simulink library "lib_rfsignalgenerator_2020a"  (R2020a)
settings: Solver=VariableStepAuto  StartTime=0.0  StopTime=10.0  RelTol=1e-3
undefined symbols (not defined in the file or in its folder): fs, QAM1024_Sym, QAM512_Sym
libraries: hdlsllib x41, simulink x15, commseqgen3 x10
(part 1 of 2)
settings Model: Creator=lewisdav  LastModifiedBy=bin
settings SFSimCC: CustomCodeUndefinedFunction=UseInterfaceOnly

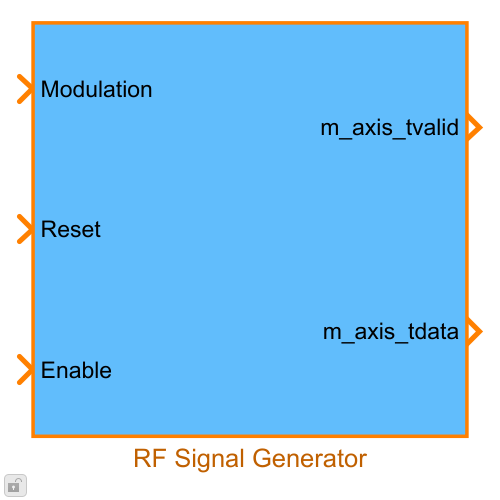
[thumbnail: Simulink's stored preview of the top-level diagram]
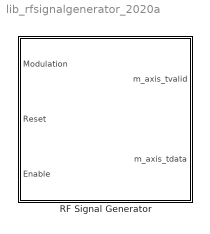
== system lib_rfsignalgenerator_2020a ==
  RF Signal Generator : Subsystem  TreatAsAtomicUnit=on

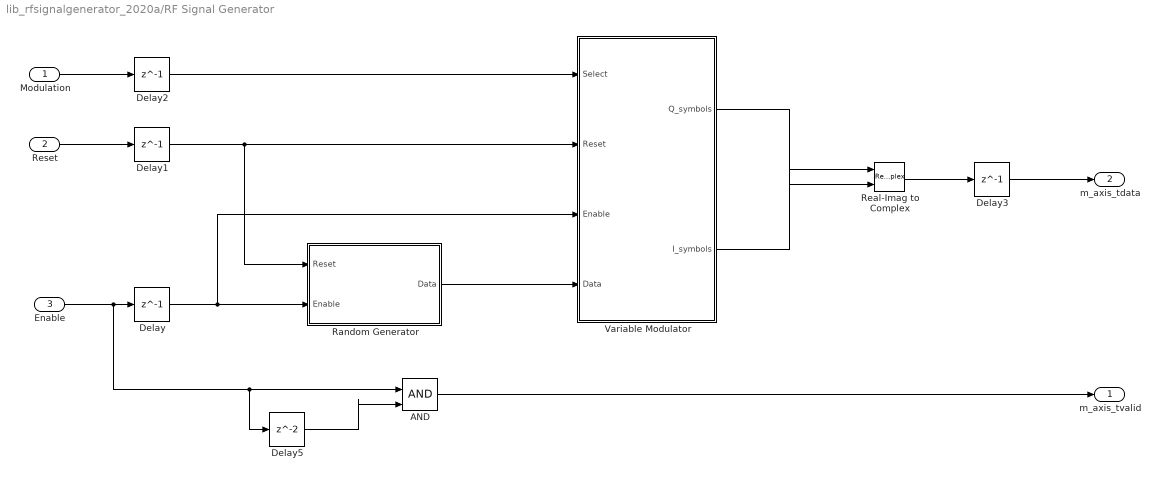
== system lib_rfsignalgenerator_2020a/RF Signal Generator ==
  Modulation : Inport
  Reset : Inport  Port=2
  Enable : Inport  Port=3
  AND : Logic  IconShape=distinctive  AllPortsSameDT=off  OutDataTypeStr=boolean
  Delay{,1..3} (4 alike) : Delay  DelayLength=1
  Delay5 : Delay
  Random Generator : Subsystem
  Real-Imag to Complex : RealImagToComplex
  Variable Modulator : Subsystem
  m_axis_tvalid : Outport  VectorParamsAs1DForOutWhenUnconnected=off
  m_axis_tdata : Outport  Port=2  VectorParamsAs1DForOutWhenUnconnected=off
  wires:
  Delay/1 -> Variable Modulator/3(Enable), Random Generator/2(Enable)
  Random Generator/1(Data) -> Variable Modulator/4(Data)
  Real-Imag to Complex/1 -> Delay3/1
  Modulation/1 -> Delay2/1
  Reset/1 -> Delay1/1
  Enable/1 -> Delay5/1, AND/1, Delay/1
  Delay1/1 -> Variable Modulator/2(Reset), Random Generator/1(Reset)
  Delay2/1 -> Variable Modulator/1(Select)
  Delay3/1 -> m_axis_tdata/1
  AND/1 -> m_axis_tvalid/1
  Variable Modulator/1(Q_symbols) -> Real-Imag to Complex/2
  Variable Modulator/2(I_symbols) -> Real-Imag to Complex/1
  Delay5/1 -> AND/2

== system lib_rfsignalgenerator_2020a/RF Signal Generator/Random Generator ==
  Reset : Inport
  Enable : Inport  Port=2
  Bit Concat1 : hdlsllib/Logic and Bit Operations/Bit Concat  numInputs=10
  Delay : Delay  DelayLength=1  ExternalReset=Level  ShowEnablePort=on  SampleTime=1/fs
      settings: InputPortMap=u0,e6,r5
  Subsystem : Subsystem
  Data : Outport  VectorParamsAs1DForOutWhenUnconnected=off
  wires:
  Enable/1 -> Subsystem/Enable, Delay/2
  Delay/1 -> Data/1
  Bit Concat1/1 -> Delay/1
  Reset/1 -> Delay/3, Subsystem/1(Reset)
  Subsystem/1(LFSR1) -> Bit Concat1/1
  Subsystem/2(LFSR2) -> Bit Concat1/2
  Subsystem/3(LFSR3) -> Bit Concat1/3
  Subsystem/4(LFSR4) -> Bit Concat1/4
  Subsystem/5(LFSR5) -> Bit Concat1/5
  Subsystem/6(LFSR6) -> Bit Concat1/6
  Subsystem/7(LFSR7) -> Bit Concat1/7
  Subsystem/8(LFSR8) -> Bit Concat1/8
  Subsystem/9(LFSR9) -> Bit Concat1/9
  Subsystem/10(LFSR10) -> Bit Concat1/10

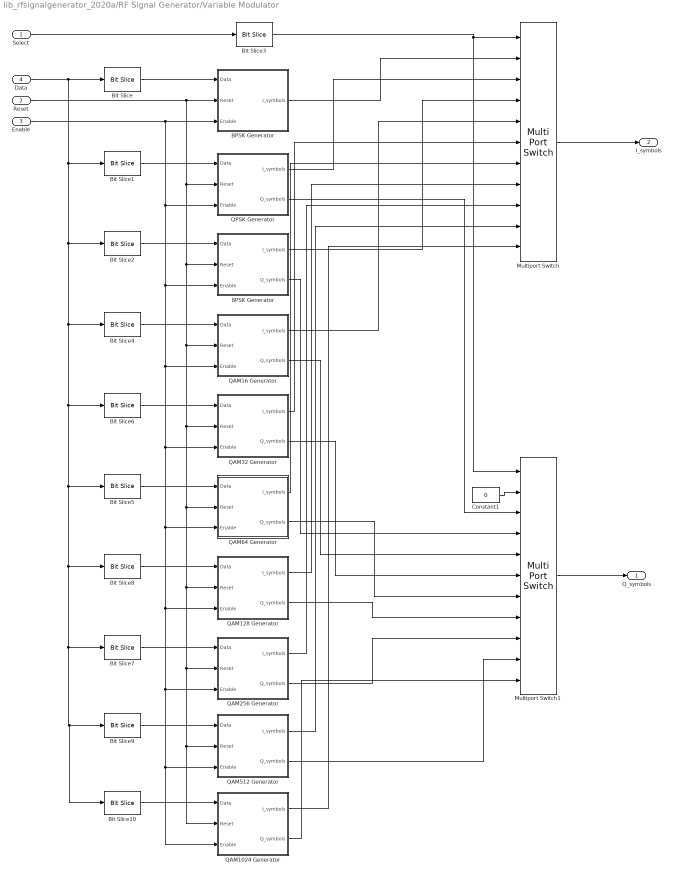
== system lib_rfsignalgenerator_2020a/RF Signal Generator/Variable Modulator ==
  Select : Inport
  Reset : Inport  Port=2
  Enable : Inport  Port=3
  Data : Inport  Port=4
  8PSK Generator : Subsystem
  BPSK Generator : Subsystem
  Bit Slice : hdlsllib/Logic and Bit Operations/Bit Slice  lidx=0  ridx=0
      settings: SourceProductBaseCode=SL
  Bit Slice1 : hdlsllib/Logic and Bit Operations/Bit Slice  lidx=1  ridx=0
      settings: SourceProductBaseCode=SL
  Bit Slice10 : hdlsllib/Logic and Bit Operations/Bit Slice  lidx=9  ridx=0
      settings: SourceProductBaseCode=SL
  Bit Slice2 : hdlsllib/Logic and Bit Operations/Bit Slice  lidx=2  ridx=0
      settings: SourceProductBaseCode=SL
  Bit Slice3 : hdlsllib/Logic and Bit Operations/Bit Slice  lidx=3  ridx=0
      settings: SourceProductBaseCode=SL
  Bit Slice4 : hdlsllib/Logic and Bit Operations/Bit Slice  lidx=3  ridx=0
      settings: SourceProductBaseCode=SL
  Bit Slice5 : hdlsllib/Logic and Bit Operations/Bit Slice  lidx=5  ridx=0
      settings: SourceProductBaseCode=SL
  Bit Slice6 : hdlsllib/Logic and Bit Operations/Bit Slice  lidx=4  ridx=0
      settings: SourceProductBaseCode=SL
  Bit Slice7 : hdlsllib/Logic and Bit Operations/Bit Slice  lidx=7  ridx=0
      settings: SourceProductBaseCode=SL
  Bit Slice8 : hdlsllib/Logic and Bit Operations/Bit Slice  lidx=6  ridx=0
      settings: SourceProductBaseCode=SL
  Bit Slice9 : hdlsllib/Logic and Bit Operations/Bit Slice  lidx=8  ridx=0
      settings: SourceProductBaseCode=SL
  Constant1 : Constant  Value=0  VectorParams1D=off  OutDataTypeStr=fixdt(0,1,0)  SampleTime=1/fs
  Multiport Switch : MultiPortSwitch  DataPortOrder=Zero-based contiguous  Inputs=10  zeroidx=on
  Multiport Switch1 : MultiPortSwitch  DataPortOrder=Zero-based contiguous  Inputs=10  zeroidx=on
  QAM1024 Generator : Subsystem
  QAM128 Generator : Subsystem
  QAM16 Generator : Subsystem
  QAM256 Generator : Subsystem
  QAM32 Generator : Subsystem
  QAM512 Generator : Subsystem
  QAM64 Generator : Subsystem
  QPSK Generator : Subsystem
  Q_symbols : Outport  VectorParamsAs1DForOutWhenUnconnected=off
  I_symbols : Outport  Port=2  VectorParamsAs1DForOutWhenUnconnected=off
  wires:
  QAM512 Generator/2(Q_symbols) -> Multiport Switch1/10
  QAM512 Generator/1(I_symbols) -> Multiport Switch/10
  Bit Slice9/1 -> QAM512 Generator/1(Data)
  Multiport Switch1/1 -> Q_symbols/1
  Multiport Switch/1 -> I_symbols/1
  QAM16 Generator/2(Q_symbols) -> Multiport Switch1/5
  QAM16 Generator/1(I_symbols) -> Multiport Switch/5
  8PSK Generator/2(Q_symbols) -> Multiport Switch1/4
  8PSK Generator/1(I_symbols) -> Multiport Switch/4
  Data/1 -> Bit Slice/1, Bit Slice1/1, Bit Slice2/1, Bit Slice5/1, Bit Slice8/1, Bit Slice7/1, Bit Slice10/1, Bit Slice9/1, Bit Slice6/1, Bit Slice4/1
  QPSK Generator/2(Q_symbols) -> Multiport Switch1/3
  QPSK Generator/1(I_symbols) -> Multiport Switch/3
  Reset/1 -> 8PSK Generator/2(Reset), QAM64 Generator/2(Reset), QAM256 Generator/2(Reset), QAM1024 Generator/2(Reset), QAM512 Generator/2(Reset), QAM128 Generator/2(Reset), QAM32 Generator/2(Reset), QAM16 Generator/2(Reset), QPSK Generator/2(Reset), BPSK Generator/2(Reset)
  Enable/1 -> BPSK Generator/3(Enable), QPSK Generator/3(Enable), 8PSK Generator/3(Enable), QAM64 Generator/3(Enable), QAM256 Generator/3(Enable), QAM1024 Generator/3(Enable), QAM512 Generator/3(Enable), QAM128 Generator/3(Enable), QAM32 Generator/3(Enable), QAM16 Generator/3(Enable)
  BPSK Generator/1(I_symbols) -> Multiport Switch/2
  Bit Slice1/1 -> QPSK Generator/1(Data)
  Select/1 -> Bit Slice3/1
  Bit Slice2/1 -> 8PSK Generator/1(Data)
  Bit Slice/1 -> BPSK Generator/1(Data)
  Constant1/1 -> Multiport Switch1/2
  Bit Slice3/1 -> Multiport Switch/1, Multiport Switch1/1
  Bit Slice4/1 -> QAM16 Generator/1(Data)
  Bit Slice5/1 -> QAM64 Generator/1(Data)
  QAM64 Generator/1(I_symbols) -> Multiport Switch/7
  QAM64 Generator/2(Q_symbols) -> Multiport Switch1/7
  Bit Slice6/1 -> QAM32 Generator/1(Data)
  QAM32 Generator/1(I_symbols) -> Multiport Switch/6
  QAM32 Generator/2(Q_symbols) -> Multiport Switch1/6
  Bit Slice7/1 -> QAM256 Generator/1(Data)
  QAM256 Generator/1(I_symbols) -> Multiport Switch/9
  QAM256 Generator/2(Q_symbols) -> Multiport Switch1/9
  Bit Slice8/1 -> QAM128 Generator/1(Data)
  QAM128 Generator/1(I_symbols) -> Multiport Switch/8
  QAM128 Generator/2(Q_symbols) -> Multiport Switch1/8
  Bit Slice10/1 -> QAM1024 Generator/1(Data)
  QAM1024 Generator/2(Q_symbols) -> Multiport Switch1/11
  QAM1024 Generator/1(I_symbols) -> Multiport Switch/11

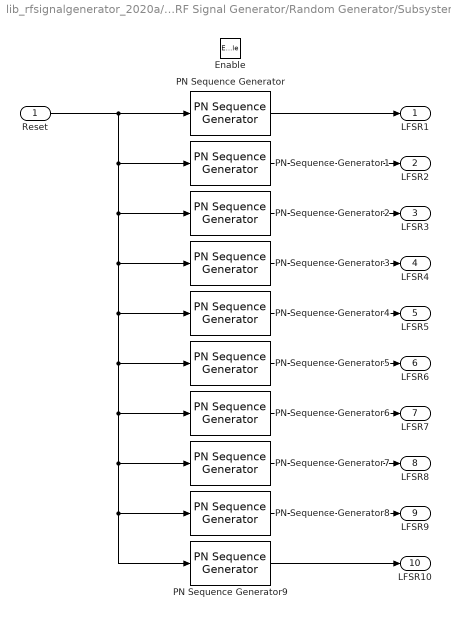
== system lib_rfsignalgenerator_2020a/RF Signal Generator/Random Generator/Subsystem ==
  Reset : Inport
  Enable : EnablePort
  PN Sequence Generator : commseqgen3/PN Sequence Generator  poly='z^13 + z^12 + z^11 + z^8 + 1'  ini_sta=[0 1 1 0 0 0 0 0 0 1 0 0 0]  outBitMaskSource=Dialog parameter  shift=0  outVarSiz=off  maxOutSizeMode=Dialog parameter  maxOutSize=[10 1]  Ts=1/fs  sampPerFrame=1  reset=on  bitPackedOutputs=off  outDataType=boolean  numPackedBits=8  bitPackDataSigned=off  bitPackedOutDType=Smallest integer
  PN Sequence Generator1 : commseqgen3/PN Sequence Generator  poly='z^13 + z^12 + z^11 + z^8 + 1'  ini_sta=[0 0 1 1 0 0 0 0 0 0 0 1 1]  outBitMaskSource=Dialog parameter  shift=0  outVarSiz=off  maxOutSizeMode=Dialog parameter  maxOutSize=[10 1]  Ts=1/fs  sampPerFrame=1  reset=on  bitPackedOutputs=off  outDataType=boolean  numPackedBits=8  bitPackDataSigned=off  bitPackedOutDType=Smallest integer
  PN Sequence Generator2 : commseqgen3/PN Sequence Generator  poly='z^13 + z^12 + z^11 + z^8 + 1'  ini_sta=[1 1 0 1 0 0 0 0 0 1 0 0 1]  outBitMaskSource=Dialog parameter  shift=0  outVarSiz=off  maxOutSizeMode=Dialog parameter  maxOutSize=[10 1]  Ts=1/fs  sampPerFrame=1  reset=on  bitPackedOutputs=off  outDataType=boolean  numPackedBits=8  bitPackDataSigned=off  bitPackedOutDType=Smallest integer
  PN Sequence Generator3 : commseqgen3/PN Sequence Generator  poly='z^13 + z^12 + z^11 + z^8 + 1'  ini_sta=[1 0 1 0 0 0 0 1 0 0 1 1 0]  outBitMaskSource=Dialog parameter  shift=0  outVarSiz=off  maxOutSizeMode=Dialog parameter  maxOutSize=[10 1]  Ts=1/fs  sampPerFrame=1  reset=on  bitPackedOutputs=off  outDataType=boolean  numPackedBits=8  bitPackDataSigned=off  bitPackedOutDType=Smallest integer
  PN Sequence Generator4 : commseqgen3/PN Sequence Generator  poly='z^13 + z^12 + z^11 + z^8 + 1'  ini_sta=[0 0 0 0 1 0 0 0 0 1 1 1 0]  outBitMaskSource=Dialog parameter  shift=0  outVarSiz=off  maxOutSizeMode=Dialog parameter  maxOutSize=[10 1]  Ts=1/fs  sampPerFrame=1  reset=on  bitPackedOutputs=off  outDataType=boolean  numPackedBits=8  bitPackDataSigned=off  bitPackedOutDType=Smallest integer
  PN Sequence Generator5 : commseqgen3/PN Sequence Generator  poly='z^13 + z^12 + z^11 + z^8 + 1'  ini_sta=[1 1 0 0 1 1 0 0 1 0 1 0 0]  outBitMaskSource=Dialog parameter  shift=0  outVarSiz=off  maxOutSizeMode=Dialog parameter  maxOutSize=[10 1]  Ts=1/fs  sampPerFrame=1  reset=on  bitPackedOutputs=off  outDataType=boolean  numPackedBits=8  bitPackDataSigned=off  bitPackedOutDType=Smallest integer
  PN Sequence Generator6 : commseqgen3/PN Sequence Generator  poly='z^13 + z^12 + z^11 + z^8 + 1'  ini_sta=[1 0 0 0 0 1 0 0 0 0 1 1 1]  outBitMaskSource=Dialog parameter  shift=0  outVarSiz=off  maxOutSizeMode=Dialog parameter  maxOutSize=[10 1]  Ts=1/fs  sampPerFrame=1  reset=on  bitPackedOutputs=off  outDataType=boolean  numPackedBits=8  bitPackDataSigned=off  bitPackedOutDType=Smallest integer
  PN Sequence Generator7 : commseqgen3/PN Sequence Generator  poly='z^13 + z^12 + z^11 + z^8 + 1'  ini_sta=[1 0 0 1 1 1 1 1 0 0 0 1 1]  outBitMaskSource=Dialog parameter  shift=0  outVarSiz=off  maxOutSizeMode=Dialog parameter  maxOutSize=[10 1]  Ts=1/fs  sampPerFrame=1  reset=on  bitPackedOutputs=off  outDataType=boolean  numPackedBits=8  bitPackDataSigned=off  bitPackedOutDType=Smallest integer
  PN Sequence Generator8 : commseqgen3/PN Sequence Generator  poly='z^13 + z^12 + z^11 + z^8 + 1'  ini_sta=[1 1 0 1 1 1 1 1 0 0 0 1 1]  outBitMaskSource=Dialog parameter  shift=0  outVarSiz=off  maxOutSizeMode=Dialog parameter  maxOutSize=[10 1]  Ts=1/fs  sampPerFrame=1  reset=on  bitPackedOutputs=off  outDataType=boolean  numPackedBits=8  bitPackDataSigned=off  bitPackedOutDType=Smallest integer
  PN Sequence Generator9 : commseqgen3/PN Sequence Generator  poly='z^13 + z^12 + z^11 + z^8 + 1'  ini_sta=[0 1 0 1 1 0 0 1 0 0 0 1 1]  outBitMaskSource=Dialog parameter  shift=0  outVarSiz=off  maxOutSizeMode=Dialog parameter  maxOutSize=[10 1]  Ts=1/fs  sampPerFrame=1  reset=on  bitPackedOutputs=off  outDataType=boolean  numPackedBits=8  bitPackDataSigned=off  bitPackedOutDType=Smallest integer
  LFSR1 : Outport  InitialOutput=0
  LFSR2 : Outport  Port=2  InitialOutput=0
  LFSR3 : Outport  Port=3  InitialOutput=0
  LFSR4 : Outport  Port=4  InitialOutput=0
  LFSR5 : Outport  Port=5  InitialOutput=0
  LFSR6 : Outport  Port=6  InitialOutput=0
  LFSR7 : Outport  Port=7  InitialOutput=0
  LFSR8 : Outport  Port=8  InitialOutput=0
  LFSR9 : Outport  Port=9  InitialOutput=0
  LFSR10 : Outport  Port=10  InitialOutput=0
  wires:
  PN Sequence Generator8/1 -> LFSR9/1
  PN Sequence Generator/1 -> LFSR1/1
  Reset/1 -> PN Sequence Generator1/1, PN Sequence Generator4/1, PN Sequence Generator5/1, PN Sequence Generator6/1, PN Sequence Generator7/1, PN Sequence Generator9/1, PN Sequence Generator8/1, PN Sequence Generator3/1, PN Sequence Generator2/1, PN Sequence Generator/1
  PN Sequence Generator3/1 -> LFSR4/1
  PN Sequence Generator4/1 -> LFSR5/1
  PN Sequence Generator1/1 -> LFSR2/1
  PN Sequence Generator2/1 -> LFSR3/1
  PN Sequence Generator5/1 -> LFSR6/1
  PN Sequence Generator6/1 -> LFSR7/1
  PN Sequence Generator7/1 -> LFSR8/1
  PN Sequence Generator9/1 -> LFSR10/1

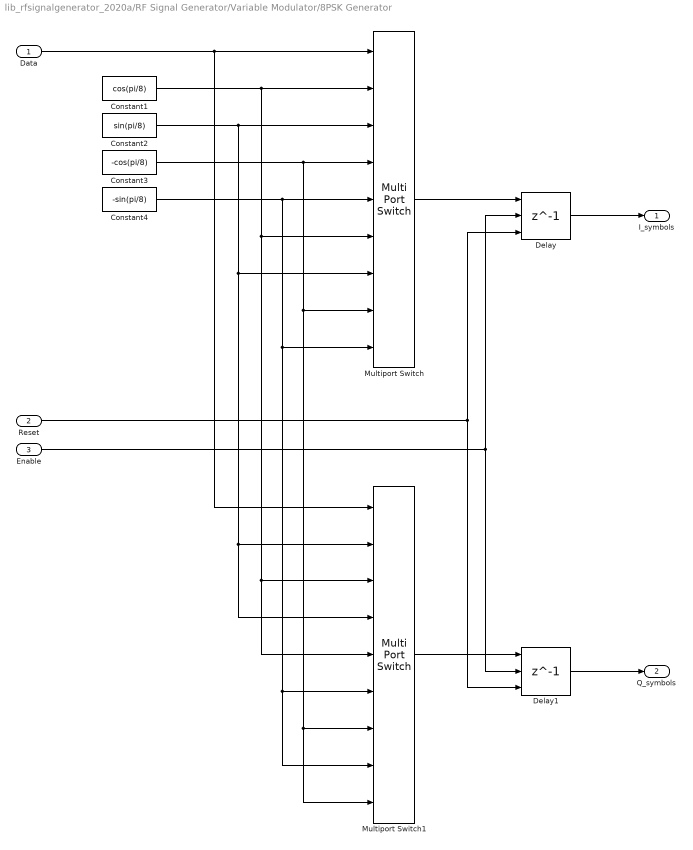
== system lib_rfsignalgenerator_2020a/RF Signal Generator/Variable Modulator/8PSK Generator ==
  Data : Inport
  Reset : Inport  Port=2
  Enable : Inport  Port=3
  Constant1 : Constant  Value=cos(pi/8)  OutDataTypeStr=fixdt(1,16,14)  SampleTime=1/fs
  Constant2 : Constant  Value=sin(pi/8)  VectorParams1D=off  OutDataTypeStr=fixdt(1,16,14)  SampleTime=1/fs
  Constant3 : Constant  Value=-cos(pi/8)  OutDataTypeStr=fixdt(1,16,14)  SampleTime=1/fs
  Constant4 : Constant  Value=-sin(pi/8)  OutDataTypeStr=fixdt(1,16,14)  SampleTime=1/fs
  Delay : Delay  DelayLength=1  ExternalReset=Level  ShowEnablePort=on  SampleTime=1/fs
      settings: InputPortMap=u0,e6,r5
  Delay1 : Delay  DelayLength=1  ExternalReset=Level  ShowEnablePort=on  SampleTime=1/fs
      settings: InputPortMap=u0,e6,r5
  Multiport Switch : MultiPortSwitch  DataPortOrder=Zero-based contiguous  Inputs=8  zeroidx=on
  Multiport Switch1 : MultiPortSwitch  DataPortOrder=Zero-based contiguous  Inputs=8  zeroidx=on
  I_symbols : Outport  VectorParamsAs1DForOutWhenUnconnected=off
  Q_symbols : Outport  Port=2  VectorParamsAs1DForOutWhenUnconnected=off
  wires:
  Delay/1 -> I_symbols/1
  Data/1 -> Multiport Switch/1, Multiport Switch1/1
  Multiport Switch/1 -> Delay/1
  Reset/1 -> Delay/3, Delay1/3
  Enable/1 -> Delay/2, Delay1/2
  Multiport Switch1/1 -> Delay1/1
  Delay1/1 -> Q_symbols/1
  Constant1/1 -> Multiport Switch1/3, Multiport Switch1/5, Multiport Switch/6, Multiport Switch/2
  Constant2/1 -> Multiport Switch1/4, Multiport Switch1/2, Multiport Switch/7, Multiport Switch/3
  Constant3/1 -> Multiport Switch1/7, Multiport Switch1/9, Multiport Switch/8, Multiport Switch/4
  Constant4/1 -> Multiport Switch1/8, Multiport Switch1/6, Multiport Switch/9, Multiport Switch/5

== system lib_rfsignalgenerator_2020a/RF Signal Generator/Variable Modulator/BPSK Generator ==
  Data : Inport
  Reset : Inport  Port=2
  Enable : Inport  Port=3
  Constant2 : Constant  OutDataTypeStr=fixdt(1,16,14)  SampleTime=1/fs
  Constant3 : Constant  Value=-1  OutDataTypeStr=fixdt(1,16,14)  SampleTime=1/fs
  Delay : Delay  DelayLength=1  InitialCondition=0  ExternalReset=Level  ShowEnablePort=on  UseCircularBuffer=on  SampleTime=1/fs
      settings: InputPortMap=u0,e6,r5
  Multiport Switch : MultiPortSwitch  DataPortOrder=Zero-based contiguous  Inputs=2  zeroidx=on
  I_symbols : Outport  VectorParamsAs1DForOutWhenUnconnected=off
  wires:
  Delay/1 -> I_symbols/1
  Enable/1 -> Delay/2
  Reset/1 -> Delay/3
  Multiport Switch/1 -> Delay/1
  Constant3/1 -> Multiport Switch/2
  Constant2/1 -> Multiport Switch/3
  Data/1 -> Multiport Switch/1

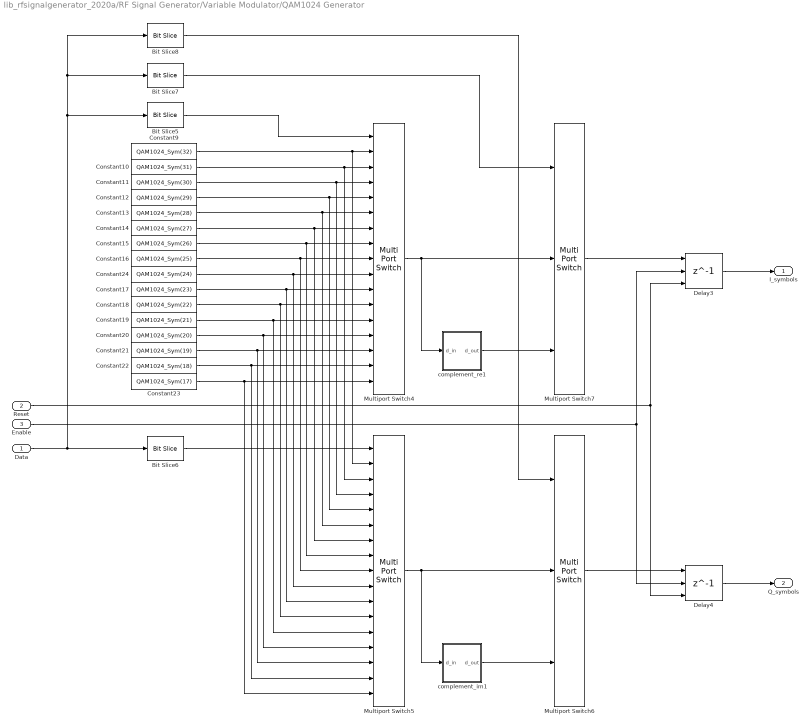
== system lib_rfsignalgenerator_2020a/RF Signal Generator/Variable Modulator/QAM1024 Generator ==
  Data : Inport
  Reset : Inport  Port=2
  Enable : Inport  Port=3
  Bit Slice5 : hdlsllib/Logic and Bit Operations/Bit Slice  lidx=3  ridx=0
      settings: SourceProductBaseCode=SL
  Bit Slice6 : hdlsllib/Logic and Bit Operations/Bit Slice  lidx=7  ridx=4
      settings: SourceProductBaseCode=SL
  Bit Slice7 : hdlsllib/Logic and Bit Operations/Bit Slice  lidx=8  ridx=8
      settings: SourceProductBaseCode=SL
  Bit Slice8 : hdlsllib/Logic and Bit Operations/Bit Slice  lidx=9  ridx=9
      settings: SourceProductBaseCode=SL
  Constant10 : Constant  Value=QAM1024_Sym(31)  OutDataTypeStr=fixdt(1,16,14)  SampleTime=1/fs
  Constant11 : Constant  Value=QAM1024_Sym(30)  OutDataTypeStr=fixdt(1,16,14)  SampleTime=1/fs
  Constant12 : Constant  Value=QAM1024_Sym(29)  OutDataTypeStr=fixdt(1,16,14)  SampleTime=1/fs
  Constant13 : Constant  Value=QAM1024_Sym(28)  OutDataTypeStr=fixdt(1,16,14)  SampleTime=1/fs
  Constant14 : Constant  Value=QAM1024_Sym(27)  OutDataTypeStr=fixdt(1,16,14)  SampleTime=1/fs
  Constant15 : Constant  Value=QAM1024_Sym(26)  OutDataTypeStr=fixdt(1,16,14)  SampleTime=1/fs
  Constant16 : Constant  Value=QAM1024_Sym(25)  OutDataTypeStr=fixdt(1,16,14)  SampleTime=1/fs
  Constant17 : Constant  Value=QAM1024_Sym(23)  OutDataTypeStr=fixdt(1,16,14)  SampleTime=1/fs
  Constant18 : Constant  Value=QAM1024_Sym(22)  OutDataTypeStr=fixdt(1,16,14)  SampleTime=1/fs
  Constant19 : Constant  Value=QAM1024_Sym(21)  OutDataTypeStr=fixdt(1,16,14)  SampleTime=1/fs
  Constant20 : Constant  Value=QAM1024_Sym(20)  OutDataTypeStr=fixdt(1,16,14)  SampleTime=1/fs
  Constant21 : Constant  Value=QAM1024_Sym(19)  OutDataTypeStr=fixdt(1,16,14)  SampleTime=1/fs
  Constant22 : Constant  Value=QAM1024_Sym(18)  OutDataTypeStr=fixdt(1,16,14)  SampleTime=1/fs
  Constant23 : Constant  Value=QAM1024_Sym(17)  OutDataTypeStr=fixdt(1,16,14)  SampleTime=1/fs
  Constant24 : Constant  Value=QAM1024_Sym(24)  OutDataTypeStr=fixdt(1,16,14)  SampleTime=1/fs
  Constant9 : Constant  Value=QAM1024_Sym(32)  OutDataTypeStr=fixdt(1,16,14)  SampleTime=1/fs
  Delay3 : Delay  DelayLength=1  ExternalReset=Level  ShowEnablePort=on  SampleTime=1/fs
      settings: InputPortMap=u0,e6,r5
  Delay4 : Delay  DelayLength=1  ExternalReset=Level  ShowEnablePort=on  SampleTime=1/fs
      settings: InputPortMap=u0,e6,r5
  Multiport Switch4 : MultiPortSwitch  DataPortOrder=Zero-based contiguous  Inputs=16  zeroidx=on
  Multiport Switch5 : MultiPortSwitch  DataPortOrder=Zero-based contiguous  Inputs=16  zeroidx=on
  Multiport Switch6 : MultiPortSwitch  DataPortOrder=Zero-based contiguous  Inputs=2  zeroidx=on
  Multiport Switch7 : MultiPortSwitch  DataPortOrder=Zero-based contiguous  Inputs=2  zeroidx=on
  complement_im1 : Subsystem
  complement_re1 : Subsystem
  I_symbols : Outport  VectorParamsAs1DForOutWhenUnconnected=off
  Q_symbols : Outport  Port=2  VectorParamsAs1DForOutWhenUnconnected=off
  wires:
  Constant9/1 -> Multiport Switch5/2, Multiport Switch4/2
  Constant10/1 -> Multiport Switch5/3, Multiport Switch4/3
  Constant11/1 -> Multiport Switch5/4, Multiport Switch4/4
  Constant13/1 -> Multiport Switch5/6, Multiport Switch4/6
  Constant12/1 -> Multiport Switch5/5, Multiport Switch4/5
  Constant14/1 -> Multiport Switch5/7, Multiport Switch4/7
  Constant15/1 -> Multiport Switch5/8, Multiport Switch4/8
  Constant16/1 -> Multiport Switch5/9, Multiport Switch4/9
  Constant23/1 -> Multiport Switch5/17, Multiport Switch4/17
  Constant22/1 -> Multiport Switch5/16, Multiport Switch4/16
  Constant21/1 -> Multiport Switch5/15, Multiport Switch4/15
  Constant19/1 -> Multiport Switch5/13, Multiport Switch4/13
  Constant18/1 -> Multiport Switch5/12, Multiport Switch4/12
  Constant17/1 -> Multiport Switch5/11, Multiport Switch4/11
  Constant24/1 -> Multiport Switch5/10, Multiport Switch4/10
  Constant20/1 -> Multiport Switch5/14, Multiport Switch4/14
  Multiport Switch5/1 -> Multiport Switch6/2, complement_im1/1(d_in)
  complement_im1/1(d_out) -> Multiport Switch6/3
  Bit Slice7/1 -> Multiport Switch7/1
  Multiport Switch4/1 -> Multiport Switch7/2, complement_re1/1(d_in)
  complement_re1/1(d_out) -> Multiport Switch7/3
  Delay3/1 -> I_symbols/1
  Delay4/1 -> Q_symbols/1
  Reset/1 -> Delay3/3, Delay4/3
  Enable/1 -> Delay3/2, Delay4/2
  Multiport Switch7/1 -> Delay3/1
  Multiport Switch6/1 -> Delay4/1
  Bit Slice5/1 -> Multiport Switch4/1
  Bit Slice6/1 -> Multiport Switch5/1
  Bit Slice8/1 -> Multiport Switch6/1
  Data/1 -> Bit Slice5/1, Bit Slice7/1, Bit Slice8/1, Bit Slice6/1

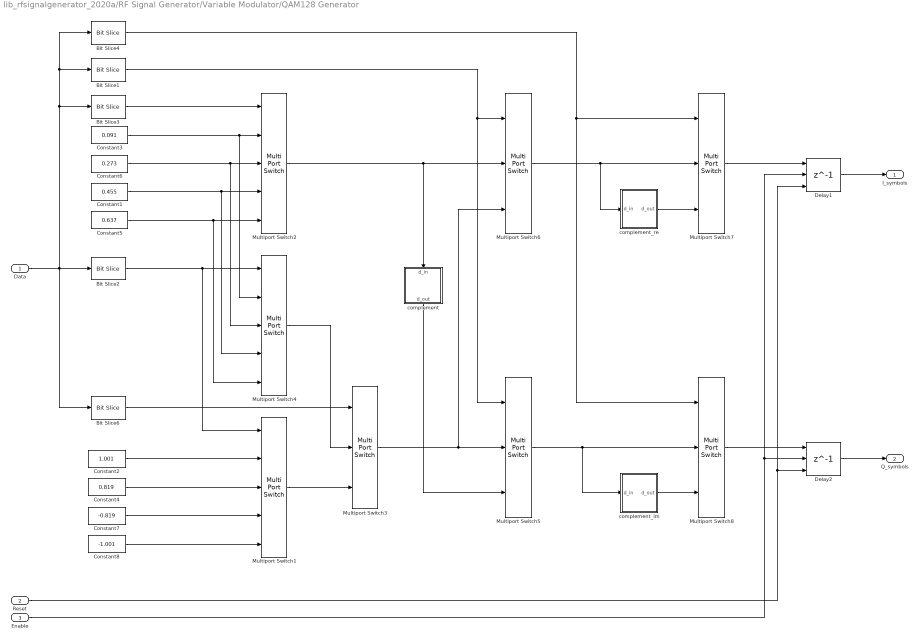
== system lib_rfsignalgenerator_2020a/RF Signal Generator/Variable Modulator/QAM128 Generator ==
  Data : Inport
  Reset : Inport  Port=2
  Enable : Inport  Port=3
  Bit Slice1 : hdlsllib/Logic and Bit Operations/Bit Slice  lidx=5  ridx=5
      settings: SourceProductBaseCode=SL
  Bit Slice2 : hdlsllib/Logic and Bit Operations/Bit Slice  lidx=3  ridx=2
      settings: SourceProductBaseCode=SL
  Bit Slice3 : hdlsllib/Logic and Bit Operations/Bit Slice  lidx=1  ridx=0
      settings: SourceProductBaseCode=SL
  Bit Slice4 : hdlsllib/Logic and Bit Operations/Bit Slice  lidx=6  ridx=6
      settings: SourceProductBaseCode=SL
  Bit Slice6 : hdlsllib/Logic and Bit Operations/Bit Slice  lidx=4  ridx=4
      settings: SourceProductBaseCode=SL
  Constant1 : Constant  Value=0.455  OutDataTypeStr=fixdt(1,16,14)  SampleTime=1/fs
  Constant2 : Constant  Value=1.001  OutDataTypeStr=fixdt(1,16,14)  SampleTime=1/fs
  Constant3 : Constant  Value=0.091  OutDataTypeStr=fixdt(1,16,14)  SampleTime=1/fs
  Constant4 : Constant  Value=0.819  OutDataTypeStr=fixdt(1,16,14)  SampleTime=1/fs
  Constant5 : Constant  Value=0.637  OutDataTypeStr=fixdt(1,16,14)  SampleTime=1/fs
  Constant6 : Constant  Value=0.273  OutDataTypeStr=fixdt(1,16,14)  SampleTime=1/fs
  Constant7 : Constant  Value=-0.819  OutDataTypeStr=fixdt(1,16,14)  SampleTime=1/fs
  Constant8 : Constant  Value=-1.001  OutDataTypeStr=fixdt(1,16,14)  SampleTime=1/fs
  Delay1 : Delay  DelayLength=1  ExternalReset=Level  ShowEnablePort=on  SampleTime=1/fs
      settings: InputPortMap=u0,e6,r5
  Delay2 : Delay  DelayLength=1  ExternalReset=Level  ShowEnablePort=on  SampleTime=1/fs
      settings: InputPortMap=u0,e6,r5
  Multiport Switch1 : MultiPortSwitch  DataPortOrder=Zero-based contiguous  Inputs=4  zeroidx=on
  Multiport Switch2 : MultiPortSwitch  DataPortOrder=Zero-based contiguous  Inputs=4  zeroidx=on
  Multiport Switch{3,5..8} (5 alike) : MultiPortSwitch  DataPortOrder=Zero-based contiguous  Inputs=2  zeroidx=on
  Multiport Switch4 : MultiPortSwitch  DataPortOrder=Zero-based contiguous  Inputs=4  zeroidx=on
  complement : Subsystem
  complement_im : Subsystem
  complement_re : Subsystem
  I_symbols : Outport  VectorParamsAs1DForOutWhenUnconnected=off
  Q_symbols : Outport  Port=2  VectorParamsAs1DForOutWhenUnconnected=off
  wires:
  Multiport Switch2/1 -> complement/1(d_in), Multiport Switch6/2
  complement/1(d_out) -> Multiport Switch5/3
  Multiport Switch3/1 -> Multiport Switch5/2, Multiport Switch6/3
  complement_re/1(d_out) -> Multiport Switch7/3
  complement_im/1(d_out) -> Multiport Switch8/3
  Bit Slice4/1 -> Multiport Switch7/1, Multiport Switch8/1
  Bit Slice1/1 -> Multiport Switch6/1, Multiport Switch5/1
  Multiport Switch8/1 -> Delay2/1
  Multiport Switch7/1 -> Delay1/1
  Multiport Switch5/1 -> complement_im/1(d_in), Multiport Switch8/2
  Multiport Switch6/1 -> complement_re/1(d_in), Multiport Switch7/2
  Bit Slice6/1 -> Multiport Switch3/1
  Multiport Switch1/1 -> Multiport Switch3/3
  Constant8/1 -> Multiport Switch1/5
  Constant7/1 -> Multiport Switch1/4
  Constant5/1 -> Multiport Switch2/5, Multiport Switch4/5
  Constant1/1 -> Multiport Switch2/4, Multiport Switch4/4
  Multiport Switch4/1 -> Multiport Switch3/2
  Data/1 -> Bit Slice3/1, Bit Slice1/1, Bit Slice4/1, Bit Slice6/1, Bit Slice2/1
  Enable/1 -> Delay1/2, Delay2/2
  Reset/1 -> Delay1/3, Delay2/3
  Constant2/1 -> Multiport Switch1/2
  Constant4/1 -> Multiport Switch1/3
  Delay2/1 -> Q_symbols/1
  Delay1/1 -> I_symbols/1
  Constant3/1 -> Multiport Switch2/2, Multiport Switch4/2
  Constant6/1 -> Multiport Switch2/3, Multiport Switch4/3
  Bit Slice3/1 -> Multiport Switch2/1
  Bit Slice2/1 -> Multiport Switch4/1, Multiport Switch1/1

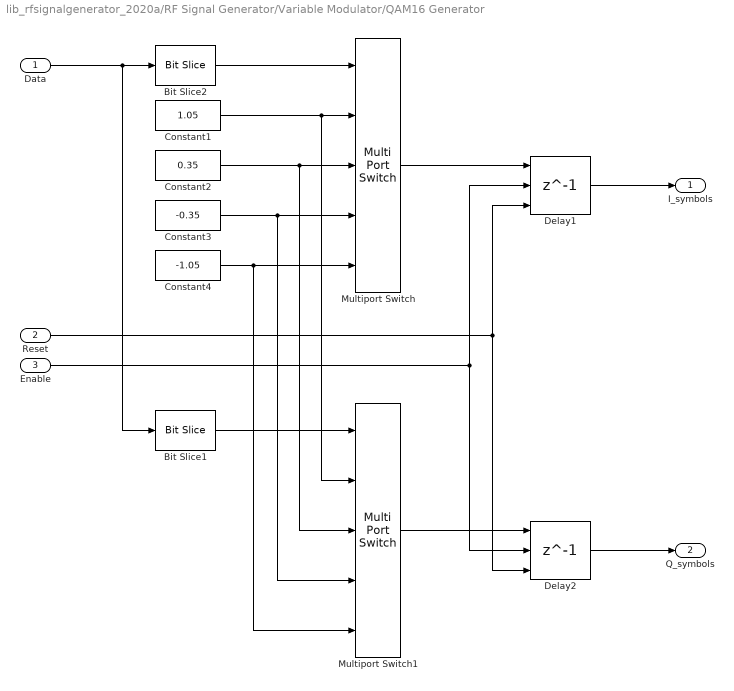
== system lib_rfsignalgenerator_2020a/RF Signal Generator/Variable Modulator/QAM16 Generator ==
  Data : Inport
  Reset : Inport  Port=2
  Enable : Inport  Port=3
  Bit Slice1 : hdlsllib/Logic and Bit Operations/Bit Slice  lidx=3  ridx=2
      settings: SourceProductBaseCode=SL
  Bit Slice2 : hdlsllib/Logic and Bit Operations/Bit Slice  lidx=1  ridx=0
      settings: SourceProductBaseCode=SL
  Constant1 : Constant  Value=1.05  OutDataTypeStr=fixdt(1,16,14)  SampleTime=1/fs
  Constant2 : Constant  Value=0.35  OutDataTypeStr=fixdt(1,16,14)  SampleTime=1/fs
  Constant3 : Constant  Value=-0.35  OutDataTypeStr=fixdt(1,16,14)  SampleTime=1/fs
  Constant4 : Constant  Value=-1.05  OutDataTypeStr=fixdt(1,16,14)  SampleTime=1/fs
  Delay1 : Delay  DelayLength=1  ExternalReset=Level  ShowEnablePort=on  SampleTime=1/fs
      settings: InputPortMap=u0,e6,r5
  Delay2 : Delay  DelayLength=1  ExternalReset=Level  ShowEnablePort=on  SampleTime=1/fs
      settings: InputPortMap=u0,e6,r5
  Multiport Switch : MultiPortSwitch  DataPortOrder=Zero-based contiguous  Inputs=4  zeroidx=on
  Multiport Switch1 : MultiPortSwitch  DataPortOrder=Zero-based contiguous  Inputs=4  zeroidx=on
  I_symbols : Outport  VectorParamsAs1DForOutWhenUnconnected=off
  Q_symbols : Outport  Port=2  VectorParamsAs1DForOutWhenUnconnected=off
  wires:
  Data/1 -> Bit Slice2/1, Bit Slice1/1
  Bit Slice2/1 -> Multiport Switch/1
  Multiport Switch/1 -> Delay1/1
  Delay1/1 -> I_symbols/1
  Multiport Switch1/1 -> Delay2/1
  Delay2/1 -> Q_symbols/1
  Reset/1 -> Delay1/3, Delay2/3
  Enable/1 -> Delay1/2, Delay2/2
  Bit Slice1/1 -> Multiport Switch1/1
  Constant1/1 -> Multiport Switch/2, Multiport Switch1/2
  Constant2/1 -> Multiport Switch/3, Multiport Switch1/3
  Constant3/1 -> Multiport Switch/4, Multiport Switch1/4
  Constant4/1 -> Multiport Switch/5, Multiport Switch1/5

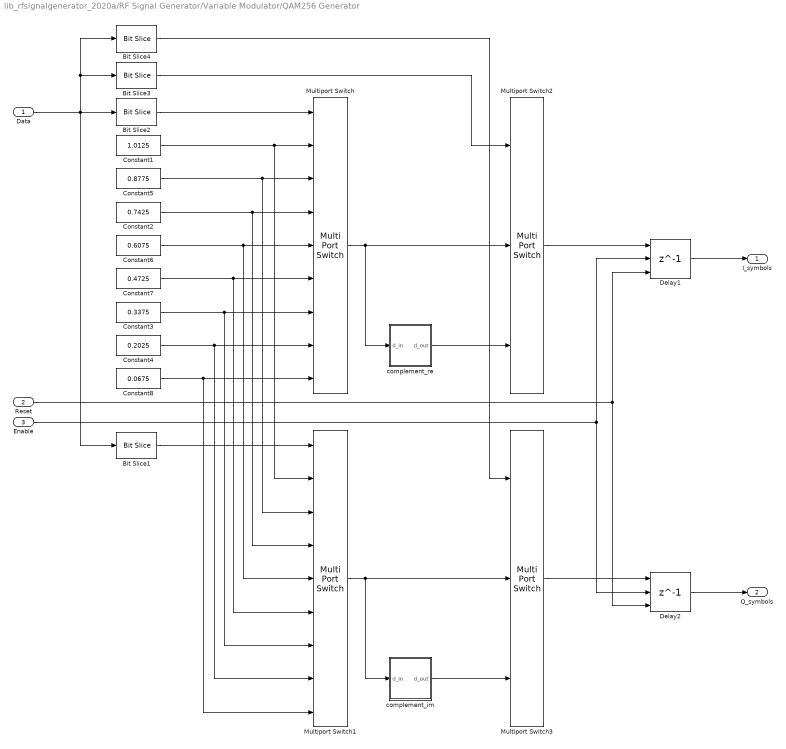
== system lib_rfsignalgenerator_2020a/RF Signal Generator/Variable Modulator/QAM256 Generator ==
  Data : Inport
  Reset : Inport  Port=2
  Enable : Inport  Port=3
  Bit Slice1 : hdlsllib/Logic and Bit Operations/Bit Slice  lidx=5  ridx=3
      settings: SourceProductBaseCode=SL
  Bit Slice2 : hdlsllib/Logic and Bit Operations/Bit Slice  lidx=2  ridx=0
      settings: SourceProductBaseCode=SL
  Bit Slice3 : hdlsllib/Logic and Bit Operations/Bit Slice  lidx=6  ridx=6
      settings: SourceProductBaseCode=SL
  Bit Slice4 : hdlsllib/Logic and Bit Operations/Bit Slice  lidx=7  ridx=7
      settings: SourceProductBaseCode=SL
  Constant1 : Constant  Value=1.0125  OutDataTypeStr=fixdt(1,16,14)  SampleTime=1/fs
  Constant2 : Constant  Value=0.7425  OutDataTypeStr=fixdt(1,16,14)  SampleTime=1/fs
  Constant3 : Constant  Value=0.3375  OutDataTypeStr=fixdt(1,16,14)  SampleTime=1/fs
  Constant4 : Constant  Value=0.2025  OutDataTypeStr=fixdt(1,16,14)  SampleTime=1/fs
  Constant5 : Constant  Value=0.8775  OutDataTypeStr=fixdt(1,16,14)  SampleTime=1/fs
  Constant6 : Constant  Value=0.6075  OutDataTypeStr=fixdt(1,16,14)  SampleTime=1/fs
  Constant7 : Constant  Value=0.4725  OutDataTypeStr=fixdt(1,16,14)  SampleTime=1/fs
  Constant8 : Constant  Value=0.0675  OutDataTypeStr=fixdt(1,16,14)  SampleTime=1/fs
  Delay1 : Delay  DelayLength=1  ExternalReset=Level  ShowEnablePort=on  SampleTime=1/fs
      settings: InputPortMap=u0,e6,r5
  Delay2 : Delay  DelayLength=1  ExternalReset=Level  ShowEnablePort=on  SampleTime=1/fs
      settings: InputPortMap=u0,e6,r5
  Multiport Switch : MultiPortSwitch  DataPortOrder=Zero-based contiguous  Inputs=8  zeroidx=on
  Multiport Switch1 : MultiPortSwitch  DataPortOrder=Zero-based contiguous  Inputs=8  zeroidx=on
  Multiport Switch2 : MultiPortSwitch  DataPortOrder=Zero-based contiguous  Inputs=2  zeroidx=on
  Multiport Switch3 : MultiPortSwitch  DataPortOrder=Zero-based contiguous  Inputs=2  zeroidx=on
  complement_im : Subsystem
  complement_re : Subsystem
  I_symbols : Outport  VectorParamsAs1DForOutWhenUnconnected=off
  Q_symbols : Outport  Port=2  VectorParamsAs1DForOutWhenUnconnected=off
  wires:
  Bit Slice1/1 -> Multiport Switch1/1
  Constant4/1 -> Multiport Switch/8, Multiport Switch1/8
  Constant7/1 -> Multiport Switch/6, Multiport Switch1/6
  Constant6/1 -> Multiport Switch/5, Multiport Switch1/5
  Constant5/1 -> Multiport Switch/3, Multiport Switch1/3
  Constant8/1 -> Multiport Switch/9, Multiport Switch1/9
  Constant3/1 -> Multiport Switch/7, Multiport Switch1/7
  Constant2/1 -> Multiport Switch/4, Multiport Switch1/4
  Data/1 -> Bit Slice2/1, Bit Slice1/1, Bit Slice4/1, Bit Slice3/1
  Bit Slice2/1 -> Multiport Switch/1
  Delay1/1 -> I_symbols/1
  Delay2/1 -> Q_symbols/1
  Reset/1 -> Delay1/3, Delay2/3
  Enable/1 -> Delay2/2, Delay1/2
  Constant1/1 -> Multiport Switch/2, Multiport Switch1/2
  Bit Slice3/1 -> Multiport Switch2/1
  Multiport Switch2/1 -> Delay1/1
  Multiport Switch3/1 -> Delay2/1
  Multiport Switch/1 -> Multiport Switch2/2, complement_re/1(d_in)
  Multiport Switch1/1 -> Multiport Switch3/2, complement_im/1(d_in)
  Bit Slice4/1 -> Multiport Switch3/1
  complement_im/1(d_out) -> Multiport Switch3/3
  complement_re/1(d_out) -> Multiport Switch2/3

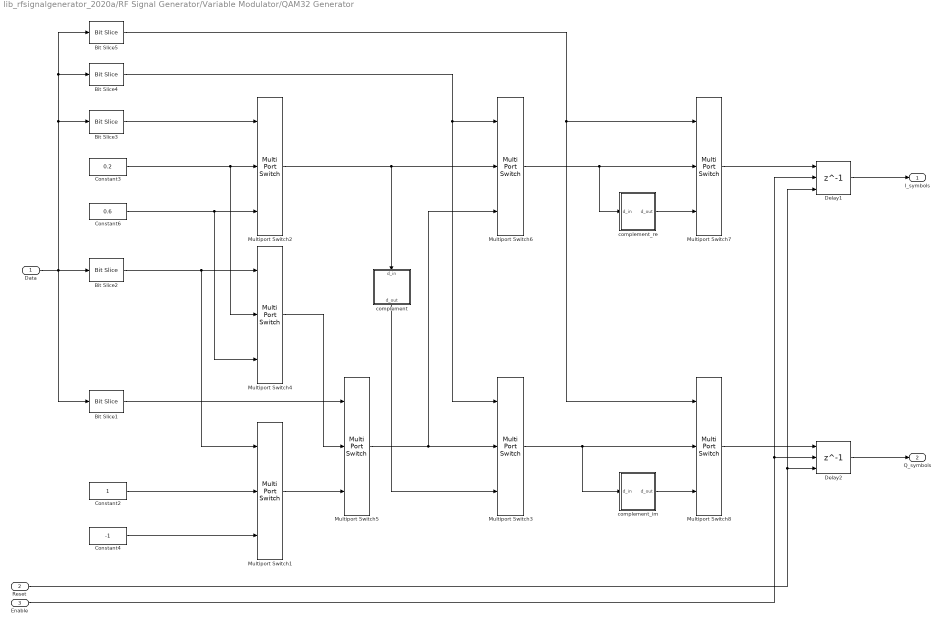
== system lib_rfsignalgenerator_2020a/RF Signal Generator/Variable Modulator/QAM32 Generator ==
  Data : Inport
  Reset : Inport  Port=2
  Enable : Inport  Port=3
  Bit Slice1 : hdlsllib/Logic and Bit Operations/Bit Slice  lidx=2  ridx=2
      settings: SourceProductBaseCode=SL
  Bit Slice2 : hdlsllib/Logic and Bit Operations/Bit Slice  lidx=1  ridx=1
      settings: SourceProductBaseCode=SL
  Bit Slice3 : hdlsllib/Logic and Bit Operations/Bit Slice  lidx=0  ridx=0
      settings: SourceProductBaseCode=SL
  Bit Slice4 : hdlsllib/Logic and Bit Operations/Bit Slice  lidx=3  ridx=3
      settings: SourceProductBaseCode=SL
  Bit Slice5 : hdlsllib/Logic and Bit Operations/Bit Slice  lidx=4  ridx=4
      settings: SourceProductBaseCode=SL
  Constant2 : Constant  OutDataTypeStr=fixdt(1,16,14)  SampleTime=1/fs
  Constant3 : Constant  Value=0.2  OutDataTypeStr=fixdt(1,16,14)  SampleTime=1/fs
  Constant4 : Constant  Value=-1  OutDataTypeStr=fixdt(1,16,14)  SampleTime=1/fs
  Constant6 : Constant  Value=0.6  OutDataTypeStr=fixdt(1,16,14)  SampleTime=1/fs
  Delay1 : Delay  DelayLength=1  ExternalReset=Level  ShowEnablePort=on  SampleTime=1/fs
      settings: InputPortMap=u0,e6,r5
  Delay2 : Delay  DelayLength=1  ExternalReset=Level  ShowEnablePort=on  SampleTime=1/fs
      settings: InputPortMap=u0,e6,r5
  Multiport Switch{1..8} (8 alike) : MultiPortSwitch  DataPortOrder=Zero-based contiguous  Inputs=2  zeroidx=on
  complement : Subsystem
  complement_im : Subsystem
  complement_re : Subsystem
  I_symbols : Outport  VectorParamsAs1DForOutWhenUnconnected=off
  Q_symbols : Outport  Port=2  VectorParamsAs1DForOutWhenUnconnected=off
  wires:
  Data/1 -> Bit Slice5/1, Bit Slice4/1, Bit Slice3/1, Bit Slice1/1, Bit Slice2/1
  Enable/1 -> Delay1/2, Delay2/2
  Reset/1 -> Delay1/3, Delay2/3
  Constant2/1 -> Multiport Switch1/2
  Constant4/1 -> Multiport Switch1/3
  Delay2/1 -> Q_symbols/1
  Delay1/1 -> I_symbols/1
  Constant3/1 -> Multiport Switch4/2, Multiport Switch2/2
  Constant6/1 -> Multiport Switch4/3, Multiport Switch2/3
  Bit Slice3/1 -> Multiport Switch2/1
  Bit Slice2/1 -> Multiport Switch1/1, Multiport Switch4/1
  Multiport Switch4/1 -> Multiport Switch5/2
  Multiport Switch1/1 -> Multiport Switch5/3
  Bit Slice4/1 -> Multiport Switch6/1, Multiport Switch3/1
  Multiport Switch5/1 -> Multiport Switch6/3, Multiport Switch3/2
  Bit Slice5/1 -> Multiport Switch8/1, Multiport Switch7/1
  Multiport Switch6/1 -> Multiport Switch7/2, complement_re/1(d_in)
  Multiport Switch3/1 -> Multiport Switch8/2, complement_im/1(d_in)
  complement/1(d_out) -> Multiport Switch3/3
  complement_re/1(d_out) -> Multiport Switch7/3
  complement_im/1(d_out) -> Multiport Switch8/3
  Multiport Switch2/1 -> Multiport Switch6/2, complement/1(d_in)
  Bit Slice1/1 -> Multiport Switch5/1
  Multiport Switch7/1 -> Delay1/1
  Multiport Switch8/1 -> Delay2/1

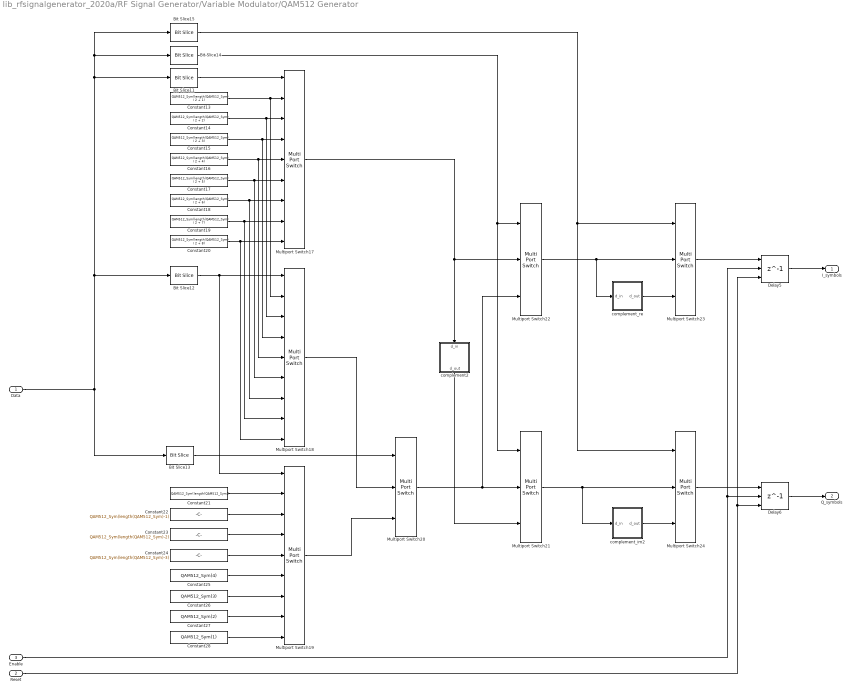
== system lib_rfsignalgenerator_2020a/RF Signal Generator/Variable Modulator/QAM512 Generator ==
  Data : Inport
  Reset : Inport  Port=2
  Enable : Inport  Port=3
  Bit Slice11 : hdlsllib/Logic and Bit Operations/Bit Slice  lidx=2  ridx=0
      settings: SourceProductBaseCode=SL
  Bit Slice12 : hdlsllib/Logic and Bit Operations/Bit Slice  lidx=5  ridx=3
      settings: SourceProductBaseCode=SL
  Bit Slice13 : hdlsllib/Logic and Bit Operations/Bit Slice  lidx=6  ridx=6
      settings: SourceProductBaseCode=SL
  Bit Slice14 : hdlsllib/Logic and Bit Operations/Bit Slice  lidx=7  ridx=7
      settings: SourceProductBaseCode=SL
  Bit Slice15 : hdlsllib/Logic and Bit Operations/Bit Slice  lidx=8  ridx=8
      settings: SourceProductBaseCode=SL
  Constant13 : Constant  Value=QAM512_Sym(length(QAM512_Sym) / 2 + 1)  OutDataTypeStr=fixdt(1,16,14)  SampleTime=1/fs
  Constant14 : Constant  Value=QAM512_Sym(length(QAM512_Sym) / 2 + 2)  OutDataTypeStr=fixdt(1,16,14)  SampleTime=1/fs
  Constant15 : Constant  Value=QAM512_Sym(length(QAM512_Sym) / 2 + 3)  OutDataTypeStr=fixdt(1,16,14)  SampleTime=1/fs
  Constant16 : Constant  Value=QAM512_Sym(length(QAM512_Sym) / 2 + 4)  OutDataTypeStr=fixdt(1,16,14)  SampleTime=1/fs
  Constant17 : Constant  Value=QAM512_Sym(length(QAM512_Sym) / 2 + 5)  OutDataTypeStr=fixdt(1,16,14)  SampleTime=1/fs
  Constant18 : Constant  Value=QAM512_Sym(length(QAM512_Sym) / 2 + 6)  OutDataTypeStr=fixdt(1,16,14)  SampleTime=1/fs
  Constant19 : Constant  Value=QAM512_Sym(length(QAM512_Sym) / 2 + 7)  OutDataTypeStr=fixdt(1,16,14)  SampleTime=1/fs
  Constant20 : Constant  Value=QAM512_Sym(length(QAM512_Sym) / 2 + 8)  OutDataTypeStr=fixdt(1,16,14)  SampleTime=1/fs
  Constant21 : Constant  Value=QAM512_Sym(length(QAM512_Sym))  OutDataTypeStr=fixdt(1,16,14)  SampleTime=1/fs
  Constant22 : Constant  Value=QAM512_Sym(length(QAM512_Sym)-1)  OutDataTypeStr=fixdt(1,16,14)  SampleTime=1/fs
  Constant23 : Constant  Value=QAM512_Sym(length(QAM512_Sym)-2)  OutDataTypeStr=fixdt(1,16,14)  SampleTime=1/fs
  Constant24 : Constant  Value=QAM512_Sym(length(QAM512_Sym)-3)  OutDataTypeStr=fixdt(1,16,14)  SampleTime=1/fs
  Constant25 : Constant  Value=QAM512_Sym(4)  OutDataTypeStr=fixdt(1,16,14)  SampleTime=1/fs
  Constant26 : Constant  Value=QAM512_Sym(3)  OutDataTypeStr=fixdt(1,16,14)  SampleTime=1/fs
  Constant27 : Constant  Value=QAM512_Sym(2)  OutDataTypeStr=fixdt(1,16,14)  SampleTime=1/fs
  Constant28 : Constant  Value=QAM512_Sym(1)  OutDataTypeStr=fixdt(1,16,14)  SampleTime=1/fs
  Delay5 : Delay  DelayLength=1  ExternalReset=Level  ShowEnablePort=on  SampleTime=1/fs
      settings: InputPortMap=u0,e6,r5
  Delay6 : Delay  DelayLength=1  ExternalReset=Level  ShowEnablePort=on  SampleTime=1/fs
      settings: InputPortMap=u0,e6,r5
  Multiport Switch17 : MultiPortSwitch  DataPortOrder=Zero-based contiguous  Inputs=8  zeroidx=on
  Multiport Switch18 : MultiPortSwitch  DataPortOrder=Zero-based contiguous  Inputs=8  zeroidx=on
  Multiport Switch19 : MultiPortSwitch  DataPortOrder=Zero-based contiguous  Inputs=8  zeroidx=on
  Multiport Switch{20..24} (5 alike) : MultiPortSwitch  DataPortOrder=Zero-based contiguous  Inputs=2  zeroidx=on
  complement2 : Subsystem
  complement_im2 : Subsystem
  complement_re : Subsystem
  I_symbols : Outport  VectorParamsAs1DForOutWhenUnconnected=off
  Q_symbols : Outport  Port=2  VectorParamsAs1DForOutWhenUnconnected=off
  wires:
  Constant13/1 -> Multiport Switch18/2, Multiport Switch17/2
  Constant14/1 -> Multiport Switch18/3, Multiport Switch17/3
  Constant15/1 -> Multiport Switch18/4, Multiport Switch17/4
  Constant16/1 -> Multiport Switch18/5, Multiport Switch17/5
  Constant17/1 -> Multiport Switch18/6, Multiport Switch17/6
  Constant18/1 -> Multiport Switch18/7, Multiport Switch17/7
  Constant19/1 -> Multiport Switch18/8, Multiport Switch17/8
  Constant20/1 -> Multiport Switch18/9, Multiport Switch17/9
  Bit Slice11/1 -> Multiport Switch17/1
  Bit Slice12/1 -> Multiport Switch19/1, Multiport Switch18/1
  Constant21/1 -> Multiport Switch19/2
  Constant22/1 -> Multiport Switch19/3
  Constant23/1 -> Multiport Switch19/4
  Constant24/1 -> Multiport Switch19/5
  Constant25/1 -> Multiport Switch19/6
  Constant26/1 -> Multiport Switch19/7
  Constant28/1 -> Multiport Switch19/9
  Constant27/1 -> Multiport Switch19/8
  Multiport Switch18/1 -> Multiport Switch20/2
  Multiport Switch19/1 -> Multiport Switch20/3
  Bit Slice13/1 -> Multiport Switch20/1
  Delay5/1 -> I_symbols/1
  Delay6/1 -> Q_symbols/1
  Reset/1 -> Delay6/3, Delay5/3
  Enable/1 -> Delay6/2, Delay5/2
  Multiport Switch22/1 -> complement_re/1(d_in), Multiport Switch23/2
  Multiport Switch21/1 -> Multiport Switch24/2, complement_im2/1(d_in)
  Multiport Switch23/1 -> Delay5/1
  Multiport Switch24/1 -> Delay6/1
  Bit Slice14/1 -> Multiport Switch21/1, Multiport Switch22/1
  Bit Slice15/1 -> Multiport Switch24/1, Multiport Switch23/1
  complement_im2/1(d_out) -> Multiport Switch24/3
  complement_re/1(d_out) -> Multiport Switch23/3
  Multiport Switch20/1 -> Multiport Switch22/3, Multiport Switch21/2
  complement2/1(d_out) -> Multiport Switch21/3
  Multiport Switch17/1 -> Multiport Switch22/2, complement2/1(d_in)
  Data/1 -> Bit Slice13/1, Bit Slice12/1, Bit Slice11/1, Bit Slice14/1, Bit Slice15/1

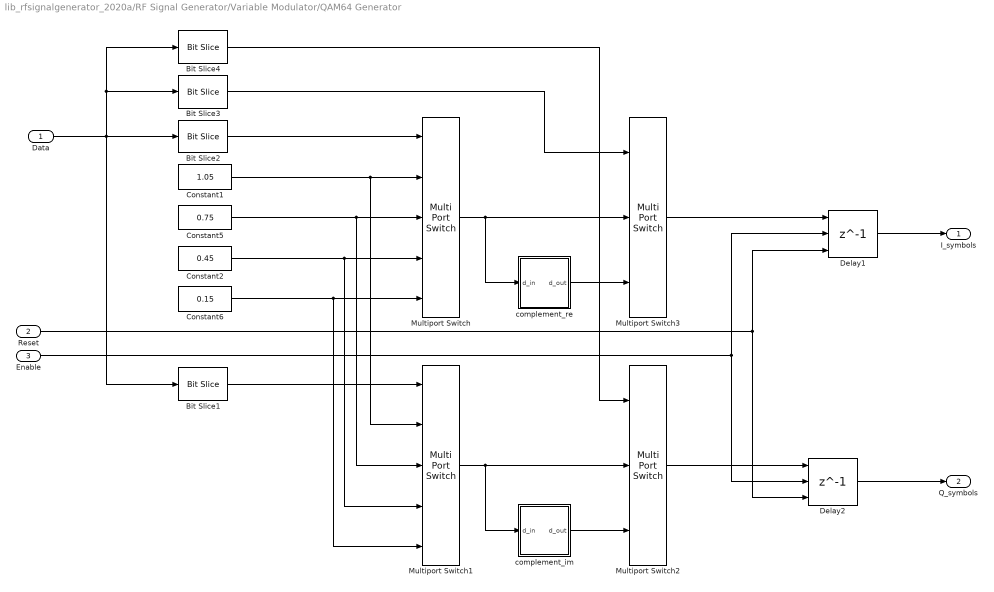
== system lib_rfsignalgenerator_2020a/RF Signal Generator/Variable Modulator/QAM64 Generator ==
  Data : Inport
  Reset : Inport  Port=2
  Enable : Inport  Port=3
  Bit Slice1 : hdlsllib/Logic and Bit Operations/Bit Slice  lidx=3  ridx=2
      settings: SourceProductBaseCode=SL
  Bit Slice2 : hdlsllib/Logic and Bit Operations/Bit Slice  lidx=1  ridx=0
      settings: SourceProductBaseCode=SL
  Bit Slice3 : hdlsllib/Logic and Bit Operations/Bit Slice  lidx=4  ridx=4
      settings: SourceProductBaseCode=SL
  Bit Slice4 : hdlsllib/Logic and Bit Operations/Bit Slice  lidx=5  ridx=5
      settings: SourceProductBaseCode=SL
  Constant1 : Constant  Value=1.05  OutDataTypeStr=fixdt(1,16,14)  SampleTime=1/fs
  Constant2 : Constant  Value=0.45  OutDataTypeStr=fixdt(1,16,14)  SampleTime=1/fs
  Constant5 : Constant  Value=0.75  OutDataTypeStr=fixdt(1,16,14)  SampleTime=1/fs
  Constant6 : Constant  Value=0.15  OutDataTypeStr=fixdt(1,16,14)  SampleTime=1/fs
  Delay1 : Delay  DelayLength=1  ExternalReset=Level  ShowEnablePort=on  SampleTime=1/fs
      settings: InputPortMap=u0,e6,r5
  Delay2 : Delay  DelayLength=1  ExternalReset=Level  ShowEnablePort=on  SampleTime=1/fs
      settings: InputPortMap=u0,e6,r5
  Multiport Switch : MultiPortSwitch  DataPortOrder=Zero-based contiguous  Inputs=4  zeroidx=on
  Multiport Switch1 : MultiPortSwitch  DataPortOrder=Zero-based contiguous  Inputs=4  zeroidx=on
  Multiport Switch2 : MultiPortSwitch  DataPortOrder=Zero-based contiguous  Inputs=2  zeroidx=on
  Multiport Switch3 : MultiPortSwitch  DataPortOrder=Zero-based contiguous  Inputs=2  zeroidx=on
  complement_im : Subsystem
  complement_re : Subsystem
  I_symbols : Outport  VectorParamsAs1DForOutWhenUnconnected=off
  Q_symbols : Outport  Port=2  VectorParamsAs1DForOutWhenUnconnected=off
  wires:
  Constant1/1 -> Multiport Switch1/2, Multiport Switch/2
  Enable/1 -> Delay1/2, Delay2/2
  Reset/1 -> Delay2/3, Delay1/3
  Delay2/1 -> Q_symbols/1
  Delay1/1 -> I_symbols/1
  Bit Slice2/1 -> Multiport Switch/1
  Data/1 -> Bit Slice1/1, Bit Slice4/1, Bit Slice3/1, Bit Slice2/1
  Constant2/1 -> Multiport Switch1/4, Multiport Switch/4
  Constant5/1 -> Multiport Switch1/3, Multiport Switch/3
  Constant6/1 -> Multiport Switch1/5, Multiport Switch/5
  Bit Slice1/1 -> Multiport Switch1/1
  complement_im/1(d_out) -> Multiport Switch2/3
  Multiport Switch1/1 -> complement_im/1(d_in), Multiport Switch2/2
  Multiport Switch/1 -> Multiport Switch3/2, complement_re/1(d_in)
  complement_re/1(d_out) -> Multiport Switch3/3
  Bit Slice3/1 -> Multiport Switch3/1
  Bit Slice4/1 -> Multiport Switch2/1
  Multiport Switch3/1 -> Delay1/1
  Multiport Switch2/1 -> Delay2/1

== system lib_rfsignalgenerator_2020a/RF Signal Generator/Variable Modulator/QPSK Generator ==
  Data : Inport
  Reset : Inport  Port=2
  Enable : Inport  Port=3
  Constant1 : Constant  Value=-0.7071  OutDataTypeStr=fixdt(1,16,14)  SampleTime=1/fs
  Constant4 : Constant  Value=0.7071  OutDataTypeStr=fixdt(1,16,14)  SampleTime=1/fs
  Delay : Delay  DelayLength=1  ExternalReset=Level  ShowEnablePort=on  SampleTime=1/fs
      settings: InputPortMap=u0,e6,r5
  Delay1 : Delay  DelayLength=1  ExternalReset=Level  ShowEnablePort=on  SampleTime=1/fs
      settings: InputPortMap=u0,e6,r5
  Multiport Switch : MultiPortSwitch  DataPortOrder=Zero-based contiguous  Inputs=4  zeroidx=on
  Multiport Switch1 : MultiPortSwitch  DataPortOrder=Zero-based contiguous  Inputs=4  zeroidx=on
  I_symbols : Outport  VectorParamsAs1DForOutWhenUnconnected=off
  Q_symbols : Outport  Port=2  VectorParamsAs1DForOutWhenUnconnected=off
  wires:
  Reset/1 -> Delay/3, Delay1/3
  Enable/1 -> Delay/2, Delay1/2
  Multiport Switch1/1 -> Delay1/1
  Delay1/1 -> Q_symbols/1
  Data/1 -> Multiport Switch/1, Multiport Switch1/1
  Multiport Switch/1 -> Delay/1
  Delay/1 -> I_symbols/1
  Constant4/1 -> Multiport Switch/2, Multiport Switch/4, Multiport Switch1/3, Multiport Switch1/2
  Constant1/1 -> Multiport Switch/3, Multiport Switch/5, Multiport Switch1/4, Multiport Switch1/5

== system lib_rfsignalgenerator_2020a/RF Signal Generator/Variable Modulator/QAM1024 Generator/complement_im1 ==
  d_in : Inport
  Add : Sum  OutDataTypeStr=uint16
  Bitwise NOT : simulink/Logic and Bit Operations/Bitwise Operator  logicop=NOT  UseBitMask=off  BitMask=bin2dec('11011001')  BitMaskRealWorld=Stored Integer
  Constant1 : Constant  OutDataTypeStr=uint16  SampleTime=1/fs
  Data Type Conversion : DataTypeConversion  OutDataTypeStr=uint16  ConvertRealWorld=Stored Integer (SI)
  Data Type Conversion1 : DataTypeConversion  OutDataTypeStr=fixdt(1,16,14)  ConvertRealWorld=Stored Integer (SI)
  d_out : Outport
  wires:
  Add/1 -> Data Type Conversion1/1
  d_in/1 -> Data Type Conversion/1
  Bitwise NOT/1 -> Add/1
  Constant1/1 -> Add/2
  Data Type Conversion/1 -> Bitwise NOT/1
  Data Type Conversion1/1 -> d_out/1

== system lib_rfsignalgenerator_2020a/RF Signal Generator/Variable Modulator/QAM1024 Generator/complement_re1 ==
  d_in : Inport
  Add : Sum  OutDataTypeStr=uint16
  Bitwise NOT : simulink/Logic and Bit Operations/Bitwise Operator  logicop=NOT  UseBitMask=off  BitMask=bin2dec('11011001')  BitMaskRealWorld=Stored Integer
  Constant1 : Constant  OutDataTypeStr=uint16  SampleTime=1/fs
  Data Type Conversion : DataTypeConversion  OutDataTypeStr=uint16  ConvertRealWorld=Stored Integer (SI)
  Data Type Conversion1 : DataTypeConversion  OutDataTypeStr=fixdt(1,16,14)  ConvertRealWorld=Stored Integer (SI)
  d_out : Outport
  wires:
  Data Type Conversion1/1 -> d_out/1
  Data Type Conversion/1 -> Bitwise NOT/1
  Constant1/1 -> Add/2
  Bitwise NOT/1 -> Add/1
  d_in/1 -> Data Type Conversion/1
  Add/1 -> Data Type Conversion1/1

== system lib_rfsignalgenerator_2020a/RF Signal Generator/Variable Modulator/QAM128 Generator/complement ==
  d_in : Inport
  Add : Sum  OutDataTypeStr=uint16
  Bitwise NOT : simulink/Logic and Bit Operations/Bitwise Operator  logicop=NOT  UseBitMask=off  BitMask=bin2dec('11011001')  BitMaskRealWorld=Stored Integer
  Constant1 : Constant  OutDataTypeStr=uint16  SampleTime=1/fs
  Data Type Conversion : DataTypeConversion  OutDataTypeStr=uint16  ConvertRealWorld=Stored Integer (SI)
  Data Type Conversion1 : DataTypeConversion  OutDataTypeStr=fixdt(1,16,14)  ConvertRealWorld=Stored Integer (SI)
  d_out : Outport
  wires:
  Add/1 -> Data Type Conversion1/1
  d_in/1 -> Data Type Conversion/1
  Bitwise NOT/1 -> Add/1
  Constant1/1 -> Add/2
  Data Type Conversion/1 -> Bitwise NOT/1
  Data Type Conversion1/1 -> d_out/1

== system lib_rfsignalgenerator_2020a/RF Signal Generator/Variable Modulator/QAM128 Generator/complement_im ==
  d_in : Inport
  Add : Sum  OutDataTypeStr=uint16
  Bitwise NOT : simulink/Logic and Bit Operations/Bitwise Operator  logicop=NOT  UseBitMask=off  BitMask=bin2dec('11011001')  BitMaskRealWorld=Stored Integer
  Constant1 : Constant  OutDataTypeStr=uint16  SampleTime=1/fs
  Data Type Conversion : DataTypeConversion  OutDataTypeStr=uint16  ConvertRealWorld=Stored Integer (SI)
  Data Type Conversion1 : DataTypeConversion  OutDataTypeStr=fixdt(1,16,14)  ConvertRealWorld=Stored Integer (SI)
  d_out : Outport
  wires:
  Add/1 -> Data Type Conversion1/1
  d_in/1 -> Data Type Conversion/1
  Bitwise NOT/1 -> Add/1
  Constant1/1 -> Add/2
  Data Type Conversion/1 -> Bitwise NOT/1
  Data Type Conversion1/1 -> d_out/1

== system lib_rfsignalgenerator_2020a/RF Signal Generator/Variable Modulator/QAM128 Generator/complement_re ==
  d_in : Inport
  Add : Sum  OutDataTypeStr=uint16
  Bitwise NOT : simulink/Logic and Bit Operations/Bitwise Operator  logicop=NOT  UseBitMask=off  BitMask=bin2dec('11011001')  BitMaskRealWorld=Stored Integer
  Constant1 : Constant  OutDataTypeStr=uint16  SampleTime=1/fs
  Data Type Conversion : DataTypeConversion  OutDataTypeStr=uint16  ConvertRealWorld=Stored Integer (SI)
  Data Type Conversion1 : DataTypeConversion  OutDataTypeStr=fixdt(1,16,14)  ConvertRealWorld=Stored Integer (SI)
  d_out : Outport
  wires:
  Data Type Conversion1/1 -> d_out/1
  Data Type Conversion/1 -> Bitwise NOT/1
  Constant1/1 -> Add/2
  Bitwise NOT/1 -> Add/1
  d_in/1 -> Data Type Conversion/1
  Add/1 -> Data Type Conversion1/1

== system lib_rfsignalgenerator_2020a/RF Signal Generator/Variable Modulator/QAM256 Generator/complement_im ==
  d_in : Inport
  Add : Sum  OutDataTypeStr=uint16
  Bitwise NOT : simulink/Logic and Bit Operations/Bitwise Operator  logicop=NOT  UseBitMask=off  BitMask=bin2dec('11011001')  BitMaskRealWorld=Stored Integer
  Constant1 : Constant  OutDataTypeStr=uint16  SampleTime=1/fs
  Data Type Conversion : DataTypeConversion  OutDataTypeStr=uint16  ConvertRealWorld=Stored Integer (SI)
  Data Type Conversion1 : DataTypeConversion  OutDataTypeStr=fixdt(1,16,14)  ConvertRealWorld=Stored Integer (SI)
  d_out : Outport
  wires:
  Add/1 -> Data Type Conversion1/1
  d_in/1 -> Data Type Conversion/1
  Bitwise NOT/1 -> Add/1
  Constant1/1 -> Add/2
  Data Type Conversion/1 -> Bitwise NOT/1
  Data Type Conversion1/1 -> d_out/1

== system lib_rfsignalgenerator_2020a/RF Signal Generator/Variable Modulator/QAM256 Generator/complement_re ==
  d_in : Inport
  Add : Sum  OutDataTypeStr=uint16
  Bitwise NOT : simulink/Logic and Bit Operations/Bitwise Operator  logicop=NOT  UseBitMask=off  BitMask=bin2dec('11011001')  BitMaskRealWorld=Stored Integer
  Constant1 : Constant  OutDataTypeStr=uint16  SampleTime=1/fs
  Data Type Conversion : DataTypeConversion  OutDataTypeStr=uint16  ConvertRealWorld=Stored Integer (SI)
  Data Type Conversion1 : DataTypeConversion  OutDataTypeStr=fixdt(1,16,14)  ConvertRealWorld=Stored Integer (SI)
  d_out : Outport
  wires:
  Data Type Conversion1/1 -> d_out/1
  Data Type Conversion/1 -> Bitwise NOT/1
  Constant1/1 -> Add/2
  Bitwise NOT/1 -> Add/1
  d_in/1 -> Data Type Conversion/1
  Add/1 -> Data Type Conversion1/1

== system lib_rfsignalgenerator_2020a/RF Signal Generator/Variable Modulator/QAM32 Generator/complement ==
  d_in : Inport
  Add : Sum  OutDataTypeStr=uint16
  Bitwise NOT : simulink/Logic and Bit Operations/Bitwise Operator  logicop=NOT  UseBitMask=off  BitMask=bin2dec('11011001')  BitMaskRealWorld=Stored Integer
  Constant1 : Constant  OutDataTypeStr=uint16  SampleTime=1/fs
  Data Type Conversion : DataTypeConversion  OutDataTypeStr=uint16  ConvertRealWorld=Stored Integer (SI)
  Data Type Conversion1 : DataTypeConversion  OutDataTypeStr=fixdt(1,16,14)  ConvertRealWorld=Stored Integer (SI)
  d_out : Outport
  wires:
  Data Type Conversion1/1 -> d_out/1
  Data Type Conversion/1 -> Bitwise NOT/1
  Constant1/1 -> Add/2
  Bitwise NOT/1 -> Add/1
  d_in/1 -> Data Type Conversion/1
  Add/1 -> Data Type Conversion1/1

== system lib_rfsignalgenerator_2020a/RF Signal Generator/Variable Modulator/QAM32 Generator/complement_im ==
  d_in : Inport
  Add : Sum  OutDataTypeStr=uint16
  Bitwise NOT : simulink/Logic and Bit Operations/Bitwise Operator  logicop=NOT  UseBitMask=off  BitMask=bin2dec('11011001')  BitMaskRealWorld=Stored Integer
  Constant1 : Constant  OutDataTypeStr=uint16  SampleTime=1/fs
  Data Type Conversion : DataTypeConversion  OutDataTypeStr=uint16  ConvertRealWorld=Stored Integer (SI)
  Data Type Conversion1 : DataTypeConversion  OutDataTypeStr=fixdt(1,16,14)  ConvertRealWorld=Stored Integer (SI)
  d_out : Outport
  wires:
  Data Type Conversion1/1 -> d_out/1
  Data Type Conversion/1 -> Bitwise NOT/1
  Constant1/1 -> Add/2
  Bitwise NOT/1 -> Add/1
  d_in/1 -> Data Type Conversion/1
  Add/1 -> Data Type Conversion1/1

== system lib_rfsignalgenerator_2020a/RF Signal Generator/Variable Modulator/QAM32 Generator/complement_re ==
  d_in : Inport
  Add : Sum  OutDataTypeStr=uint16
  Bitwise NOT : simulink/Logic and Bit Operations/Bitwise Operator  logicop=NOT  UseBitMask=off  BitMask=bin2dec('11011001')  BitMaskRealWorld=Stored Integer
  Constant1 : Constant  OutDataTypeStr=uint16  SampleTime=1/fs
  Data Type Conversion : DataTypeConversion  OutDataTypeStr=uint16  ConvertRealWorld=Stored Integer (SI)
  Data Type Conversion1 : DataTypeConversion  OutDataTypeStr=fixdt(1,16,14)  ConvertRealWorld=Stored Integer (SI)
  d_out : Outport
  wires:
  Add/1 -> Data Type Conversion1/1
  d_in/1 -> Data Type Conversion/1
  Bitwise NOT/1 -> Add/1
  Constant1/1 -> Add/2
  Data Type Conversion/1 -> Bitwise NOT/1
  Data Type Conversion1/1 -> d_out/1

== system lib_rfsignalgenerator_2020a/RF Signal Generator/Variable Modulator/QAM512 Generator/complement2 ==
  d_in : Inport
  Add : Sum  OutDataTypeStr=uint16
  Bitwise NOT : simulink/Logic and Bit Operations/Bitwise Operator  logicop=NOT  UseBitMask=off  BitMask=bin2dec('11011001')  BitMaskRealWorld=Stored Integer
  Constant1 : Constant  OutDataTypeStr=uint16  SampleTime=1/fs
  Data Type Conversion : DataTypeConversion  OutDataTypeStr=uint16  ConvertRealWorld=Stored Integer (SI)
  Data Type Conversion1 : DataTypeConversion  OutDataTypeStr=fixdt(1,16,14)  ConvertRealWorld=Stored Integer (SI)
  d_out : Outport
  wires:
  Add/1 -> Data Type Conversion1/1
  d_in/1 -> Data Type Conversion/1
  Bitwise NOT/1 -> Add/1
  Constant1/1 -> Add/2
  Data Type Conversion/1 -> Bitwise NOT/1
  Data Type Conversion1/1 -> d_out/1
